simulink model "MGietka_1d"  (R2020b)
settings: Solver=VariableStepAuto  StartTime=0.0  StopTime=10.0  RelTol=1e-3
settings Model: Creator=Mati  LastModifiedBy=Mati

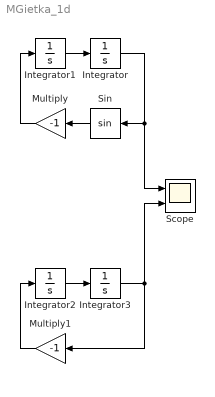
== system MGietka_1d ==
  Integrator : Integrator  InitialCondition=1
  Integrator1 : Integrator
  Integrator2 : Integrator
  Integrator3 : Integrator  InitialCondition=1
  Multiply : Gain  Gain=-1
  Multiply1 : Gain  Gain=-1
  Scope : Scope  NumInputPorts=2
  Sin : Trigonometry
  wires:
  Integrator2/1 -> Integrator3/1
  Integrator1/1 -> Integrator/1
  Sin/1 -> Multiply/1
  Multiply1/1 -> Integrator2/1
  Multiply/1 -> Integrator1/1
  Integrator/1 -> Sin/1, Scope/1
  Integrator3/1 -> Multiply1/1, Scope/2
